simulink library "cdsEpicsOutInt"  (Simulink 6.2)
settings Model: LastModifiedBy=rolf

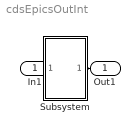
== system cdsEpicsOutInt ==
  In1 : Inport  Port=1  LatchInput=off
  Subsystem : Subsystem
  Out1 : Outport
  wires:
  Subsystem/1(Out1) -> Out1/1
  In1/1 -> Subsystem/1(In1)

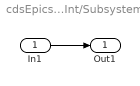
== system cdsEpicsOutInt/Subsystem ==
  In1 : Inport  Port=1  LatchInput=off
  Out1 : Outport
  wires:
  In1/1 -> Out1/1
